simulink model "gmStateSpaceHDL_buck_convert_test1_fixpt"  (R2025a)
settings: Solver=FixedStepAuto  StartTime=0.0  StopTime=0.0005  FixedStep=25e-9  RelTol=1e-3  AbsTol=1e-3
InitFcn:
  | load('C:\Users\bensa\Desktop\PI3_FPGA_BuckConverter\sschdl\buck_convert_test1\stateSpaceParameters.mat');
model workspace (MAT data in the model file):
  NoaFutureIOMap{1}.PortName = 'rst'
  NoaFutureIOMap{1}.PortType = 'Inport'
  NoaFutureIOMap{1}.DataType = 'uint32'
  NoaFutureIOMap{1}.IOInterface = 'AXI4-Lite'
  NoaFutureIOMap{1}.IOInterfaceMapping = 'x"100"'
  NoaFutureIOMap{2}.PortName = 'duty_open_loop'
  NoaFutureIOMap{2}.PortType = 'Inport'
  NoaFutureIOMap{2}.DataType = 'uint32'
  NoaFutureIOMap{2}.IOInterface = 'AXI4-Lite'
  NoaFutureIOMap{2}.IOInterfaceMapping = 'x"104"'
  NoaFutureIOMap{3}.PortName = 'freq'
  NoaFutureIOMap{3}.PortType = 'Inport'
  NoaFutureIOMap{3}.DataType = 'uint32'
  NoaFutureIOMap{3}.IOInterface = 'AXI4-Lite'
  NoaFutureIOMap{3}.IOInterfaceMapping = 'x"108"'
  NoaFutureIOMap{4}.PortName = 'en'
  NoaFutureIOMap{4}.PortType = 'Inport'
  NoaFutureIOMap{4}.DataType = 'uint32'
  NoaFutureIOMap{4}.IOInterface = 'AXI4-Lite'
  NoaFutureIOMap{4}.IOInterfaceMapping = 'x"10C"'
  NoaFutureIOMap{5}.PortName = 'mode_controller'
  NoaFutureIOMap{5}.PortType = 'Inport'
  NoaFutureIOMap{5}.DataType = 'uint32'
  NoaFutureIOMap{5}.IOInterface = 'AXI4-Lite'
  NoaFutureIOMap{5}.IOInterfaceMapping = 'x"110"'
  NoaFutureIOMap{6}.PortName = 'vout_ref'
  NoaFutureIOMap{6}.PortType = 'Inport'
  NoaFutureIOMap{6}.DataType = 'uint32'
  NoaFutureIOMap{6}.IOInterface = 'AXI4-Lite'
  NoaFutureIOMap{6}.IOInterfaceMapping = 'x"114"'
  NoaFutureIOMap{7}.PortName = 'vin'
  NoaFutureIOMap{7}.PortType = 'Outport'
  NoaFutureIOMap{7}.DataType = 'sfix32_En27'
  NoaFutureIOMap{7}.IOInterface = 'DAQ Channel 1 [0:31]'
  NoaFutureIOMap{7}.IOInterfaceMapping = '[0:31]'
  NoaFutureIOMap{8}.PortName = 'vout'
  NoaFutureIOMap{8}.PortType = 'Outport'
  NoaFutureIOMap{8}.DataType = 'sfix32_En27'
  NoaFutureIOMap{8}.IOInterface = 'DAQ Channel 0 [0:31]'
  NoaFutureIOMap{8}.IOInterfaceMapping = '[0:31]'
  NoaFutureIOMap{9}.PortName = 'vout_analog'
  NoaFutureIOMap{9}.PortType = 'Outport'
  NoaFutureIOMap{9}.DataType = 'sfix32_En27'
  NoaFutureIOMap{9}.IOInterface = 'Analog Output 0 [0:31]'
  NoaFutureIOMap{9}.IOInterfaceMapping = '[0:31]'
  NoaFutureIOMap{9}.NoaBlockParameters.SignalMin = '0'
  NoaFutureIOMap{9}.NoaBlockParameters.SignalMax = '12'
  NoaFutureIOMap{9}.NoaBlockParameters.VoltageMin = '0'
  NoaFutureIOMap{9}.NoaBlockParameters.VoltageMax = '4'
  NoaFutureIOMap{9}.NoaBlockParameters.LUT_Signals = '[0          1.2          2.4          3.6          4.8            6          7.2          8.4          9.6         10.8           12]'
  NoaFutureIOMap{9}.NoaBlockParameters.LUT_Values = '[0         0.4         0.8         1.2         1.6           2         2.4         2.8         3.2         3.6           4]'
  NoaFutureIOMap{10}.PortName = 'pwm'
  NoaFutureIOMap{10}.PortType = 'Outport'
  NoaFutureIOMap{10}.DataType = 'ufix32_En29'
  NoaFutureIOMap{10}.IOInterface = 'DAQ Channel 2 [0:31]'
  NoaFutureIOMap{10}.IOInterfaceMapping = '[0:31]'
  NoaFutureIOMap{11}.PortName = 'error_controller'
  NoaFutureIOMap{11}.PortType = 'Outport'
  NoaFutureIOMap{11}.DataType = 'sfix32_En25'
  NoaFutureIOMap{11}.IOInterface = 'DAQ Channel 3 [0:31]'
  NoaFutureIOMap{11}.IOInterfaceMapping = '[0:31]'
values from neighbouring files (symbols this model uses):
  stateSpaceParameters_1 =     [stateSpaceParameters.mat]
libraries: hdlsllib x4, hdlssclib x4, library_AnalogOut x1, simulink x1
CloseFcn:
  | clear stateSpaceParameters_1
settings Model: MinMaxOverflowLogging=MinMaxAndOverflow  FPTRunName=EmbeddedRun1  Creator=bensa  LastModifiedBy=bensa
settings SolverCC: AutoScaleAbsTol=off  AlgebraicLoopSolver=TrustRegion  AutoInsertRateTranBlk=on  MaxZcPerStep=1.0
settings OptimizationCC: BlockReduction=off  ConditionallyExecuteInputs=off  DefaultParameterBehavior=Inlined  InheritOutputTypeSmallerThanSingle=on
settings DebuggingCC: SignalRangeChecking=warning  ArtificialAlgebraicLoopMsg=error  SingleTaskRateTransMsg=error  ParameterOverflowMsg=warning  ParameterUnderflowMsg=warning  UnconnectedInputMsg=warning  UnconnectedOutputMsg=warning  UnconnectedLineMsg=warning  SymbolicDimsDataTypeCodeGenerationDiagnostic=none
settings HardwareCC: ProdBitPerPointer=32.0  ProdBitPerSizeT=32.0  ProdBitPerPtrDiffT=32.0  ProdLargestAtomicFloat=None  ProdIntDivRoundTo=Undefined  ProdEndianess=Unspecified  ProdWordSize=32.0  ProdHWDeviceType=ASIC/FPGA->ASIC/FPGA  TargetBitPerPointer=64.0  TargetBitPerSizeT=64.0  TargetBitPerPtrDiffT=64.0  TargetLongLongMode=on  TargetIntDivRoundTo=Zero  TargetEndianess=LittleEndian  TargetWordSize=64.0  TargetHWDeviceType=Custom Processor->MATLAB Host Computer  ProdEqTarget=off
settings ModelReferenceCC: EnableRefExpFcnMdlSchedulingChecks=on
settings SFSimCC: CustomCodeUndefinedFunction=UseInterfaceOnly
settings RTWCC: GPUComputeCapability=3.5  DLArmComputeVersion=19.05
settings SimscapeCC: SimscapeLogType=all  SimscapeLogSimulationStatistics=on  SimscapeLogDataHistory=10000.0

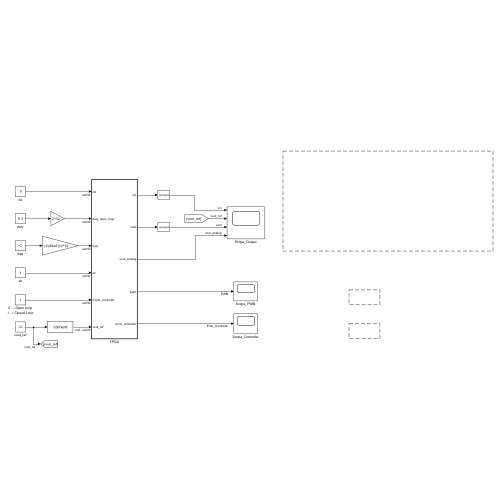
[thumbnail: Simulink's stored preview of the top-level diagram]
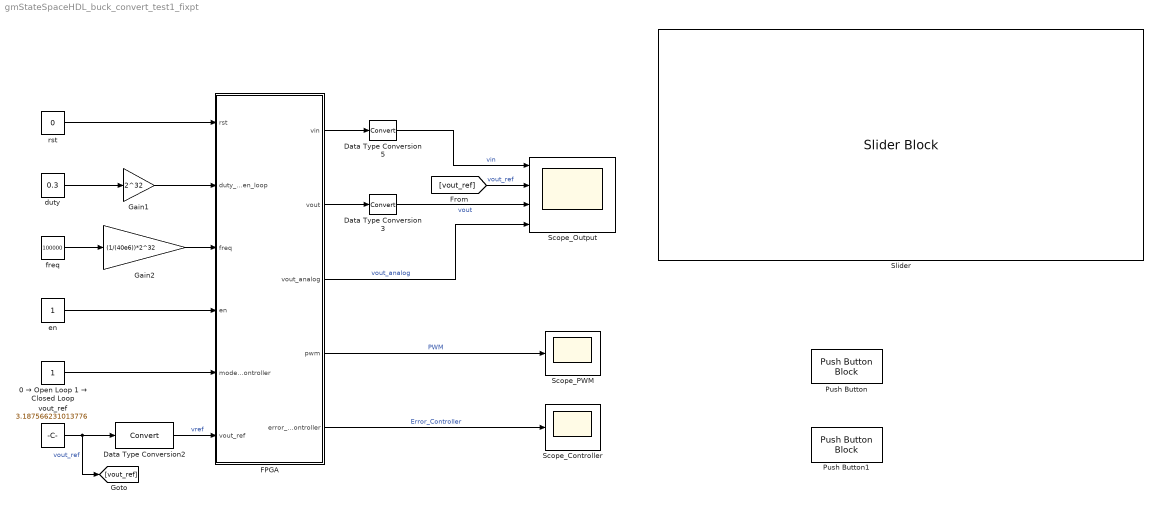
== system gmStateSpaceHDL_buck_convert_test1_fixpt ==
  0 → Open Loop 1 → Closed Loop : Constant  OutDataTypeStr=uint32  SampleTime=25e-9
  Data Type Conversion2 : DataTypeConversion  SaturateOnIntegerOverflow=off  RndMeth=Floor
  Data Type Conversion3 : DataTypeConversion  RndMeth=Nearest  SaturateOnIntegerOverflow=off  LockScale=on
  Data Type Conversion5 : DataTypeConversion  RndMeth=Nearest  SaturateOnIntegerOverflow=off  LockScale=on
  FPGA : Subsystem  TreatAsAtomicUnit=on
  Gain1 : Gain  Gain=2^32  OutDataTypeStr=uint32
  Gain2 : Gain  Gain=(1/(40e6))*2^32  OutDataTypeStr=uint32
  Push Button : PushButtonBlock  IconOnColor=[0.0, 0.39215686274509803, 0.0]  IconOffColor=[0.0, 1.0, 0.0]
  Push Button1 : PushButtonBlock  IconOnColor=[0.0, 0.39215686274509803, 0.0]  IconOffColor=[0.0, 1.0, 0.0]
  Scope_Controller : Scope
      settings: ActiveDisplayYMinimum=-13.875  ActiveDisplayYMaximum=24.875  DataLoggingVariableName=ScopeData3
  Scope_Output : Scope  NumInputPorts=4
      settings: ActiveDisplayYMinimum=-1.4999999999999996  ActiveDisplayYMaximum=13.5
  Scope_PWM : Scope
      settings: ActiveDisplayYMinimum=-0.62499999999999989  ActiveDisplayYMaximum=5.625
  Slider : SliderBlock  LabelPosition=Bottom  ScaleMax=12
  duty : Constant  Value=0.3  OutDataTypeStr=double  SampleTime=25e-9
  en : Constant  OutDataTypeStr=uint32  SampleTime=25e-9
  freq : Constant  Value=100000  SampleTime=25e-9
  rst : Constant  Value=0  OutDataTypeStr=uint32  SampleTime=25e-9
  vout_ref : Constant  Value=3.187566231013776  OutDataTypeStr=double  SampleTime=25e-9
  wires:
  rst/1 -> FPGA/1(rst)
  0 → Open Loop 1 → Closed Loop/1 -> FPGA/5(mode_controller)
  duty/1 -> Gain1/1
  en/1 -> FPGA/4(en)
  Gain2/1 -> FPGA/3(freq)
  vout_ref/1 -> [vout_ref], Data Type Conversion2/1  "vout_ref"
  Gain1/1 -> FPGA/2(duty_open_loop)
  Data Type Conversion2/1 -> FPGA/6(vout_ref)  "vref"
  FPGA/1(vin) -> Data Type Conversion5/1
  FPGA/2(vout) -> Data Type Conversion3/1
  Data Type Conversion5/1 -> Scope_Output/1  "vin"
  [vout_ref] -> Scope_Output/2  "vout_ref"
  Data Type Conversion3/1 -> Scope_Output/3  "vout"
  FPGA/3(vout_analog) -> Scope_Output/4  "vout_analog"
  FPGA/5(error_controller) -> Scope_Controller/1  "Error_Controller"
  FPGA/4(pwm) -> Scope_PWM/1  "PWM"
  freq/1 -> Gain2/1

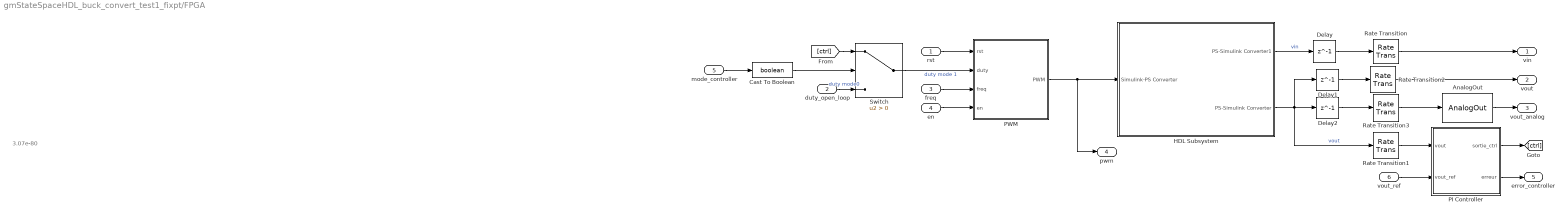
== system gmStateSpaceHDL_buck_convert_test1_fixpt/FPGA ==
  note: 3.07e-80
  rst : Inport  OutDataTypeStr=uint32
  duty_open_loop : Inport  Port=2  OutDataTypeStr=uint32
  freq : Inport  Port=3  OutDataTypeStr=uint32
  en : Inport  Port=4  OutDataTypeStr=uint32
  mode_controller : Inport  Port=5  OutDataTypeStr=uint32
  vout_ref : Inport  Port=6  OutDataTypeStr=uint32
  AnalogOut : library_AnalogOut/AnalogOut  SignalMin=0  SignalMax=12  VoltageMin=0  VoltageMax=4
  Cast To Boolean : DataTypeConversion  OutDataTypeStr=boolean  SaturateOnIntegerOverflow=off  RndMeth=Floor
  Delay : Delay  DelayLength=1
  Delay1 : Delay  DelayLength=1
  Delay2 : Delay  DelayLength=1
  HDL Subsystem : Subsystem  DataTypeOverride=Off  MinMaxOverflowLogging=MinMaxAndOverflow
  PI Controller : Subsystem
  PWM : Subsystem
  Rate Transition : RateTransition  OutPortSampleTime=25e-9
  Rate Transition1 : RateTransition
  Rate Transition2 : RateTransition  OutPortSampleTime=25e-9
  Rate Transition3 : RateTransition  OutPortSampleTime=25e-9
  Switch : Switch  Criteria=u2 > Threshold  SaturateOnIntegerOverflow=off  InputSameDT=off
  vin : Outport
  vout : Outport  Port=2
  vout_analog : Outport  Port=3
  pwm : Outport  Port=4
  error_controller : Outport  Port=5
  wires:
  en/1 -> PWM/4(en)
  mode_controller/1 -> Cast To Boolean/1
  rst/1 -> PWM/1(rst)
  freq/1 -> PWM/3(freq)
  Cast To Boolean/1 -> Switch/2
  Switch/1 -> PWM/2(duty)  "duty mode 1"
  PWM/1(PWM) -> pwm/1, HDL Subsystem/1(Simulink-PS Converter)
  HDL Subsystem/1(PS-Simulink Converter1) -> Delay/1  "vin"
  HDL Subsystem/2(PS-Simulink Converter) -> Rate Transition1/1, Delay2/1, Delay1/1  "vout"
  Delay1/1 -> Rate Transition2/1
  Delay/1 -> Rate Transition/1
  Rate Transition2/1 -> vout/1
  Rate Transition/1 -> vin/1
  AnalogOut/1 -> vout_analog/1
  duty_open_loop/1 -> Switch/3  "duty mode0"
  vout_ref/1 -> PI Controller/2(vout_ref)
  PI Controller/2(erreur) -> error_controller/1
  Rate Transition1/1 -> PI Controller/1(vout)
  Delay2/1 -> Rate Transition3/1
  Rate Transition3/1 -> AnalogOut/1
  PI Controller/1(sortie_ctrl) -> [ctrl]
  [ctrl] -> Switch/1

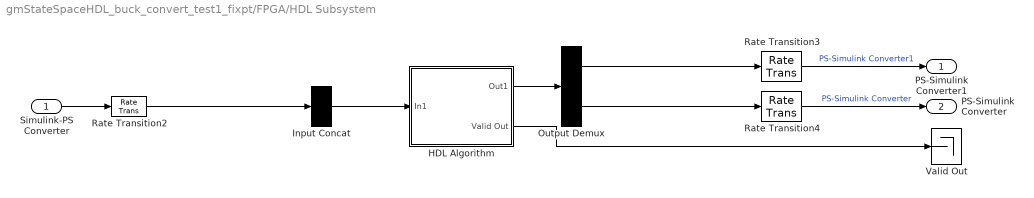
== system gmStateSpaceHDL_buck_convert_test1_fixpt/FPGA/HDL Subsystem ==
  Simulink-PS Converter : Inport  OutDataTypeStr=fixdt(0,32,29)
  HDL Algorithm : Subsystem
  Input Concat : Concatenate  NumInputs=1
  Output Demux : Demux  Outputs=2
  Rate Transition2 : RateTransition  Integrity=off  OutPortSampleTimeOpt=Multiple of input port sample time  OutPortSampleTimeMultiple=1/2
  Rate Transition3 : RateTransition  OutPortSampleTimeOpt=Multiple of input port sample time  OutPortSampleTimeMultiple=2
  Rate Transition4 : RateTransition  OutPortSampleTimeOpt=Multiple of input port sample time  OutPortSampleTimeMultiple=2
  Valid Out : Terminator
  PS-Simulink Converter1 : Outport
  PS-Simulink Converter : Outport  Port=2
  wires:
  Output Demux/2 -> Rate Transition4/1
  Rate Transition3/1 -> PS-Simulink Converter1/1  "PS-Simulink Converter1"
  HDL Algorithm/2(Valid Out) -> Valid Out/1
  Input Concat/1 -> HDL Algorithm/1(In1)
  Output Demux/1 -> Rate Transition3/1
  Simulink-PS Converter/1 -> Rate Transition2/1
  HDL Algorithm/1(Out1) -> Output Demux/1
  Rate Transition4/1 -> PS-Simulink Converter/1  "PS-Simulink Converter"
  Rate Transition2/1 -> Input Concat/1

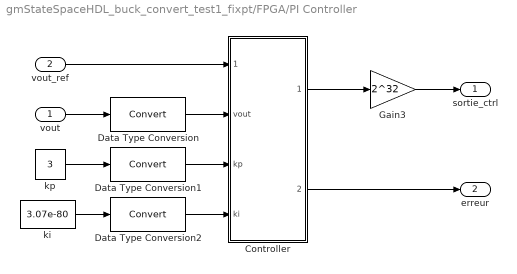
== system gmStateSpaceHDL_buck_convert_test1_fixpt/FPGA/PI Controller ==
  vout : Inport
  vout_ref : Inport  Port=2  OutDataTypeStr=uint32
  Controller : Subsystem
  Data Type Conversion : DataTypeConversion  SaturateOnIntegerOverflow=off  RndMeth=Floor
  Data Type Conversion1 : DataTypeConversion  SaturateOnIntegerOverflow=off  RndMeth=Floor
  Data Type Conversion2 : DataTypeConversion  SaturateOnIntegerOverflow=off  RndMeth=Floor
  Gain3 : Gain  Gain=2^32  OutDataTypeStr=uint32
  ki : Constant  Value=3.07e-80  OutDataTypeStr=double  SampleTime=25e-9
  kp : Constant  Value=3  OutDataTypeStr=double  SampleTime=25e-9
  sortie_ctrl : Outport
  erreur : Outport  Port=2
  wires:
  vout/1 -> Data Type Conversion/1
  Controller/1(sortie_ctrl) -> Gain3/1
  Data Type Conversion1/1 -> Controller/3(kp)
  kp/1 -> Data Type Conversion1/1
  ki/1 -> Data Type Conversion2/1
  vout_ref/1 -> Controller/1(vout_ref)
  Data Type Conversion/1 -> Controller/2(vout)
  Data Type Conversion2/1 -> Controller/4(ki)
  Gain3/1 -> sortie_ctrl/1
  Controller/2(error_ctrl) -> erreur/1

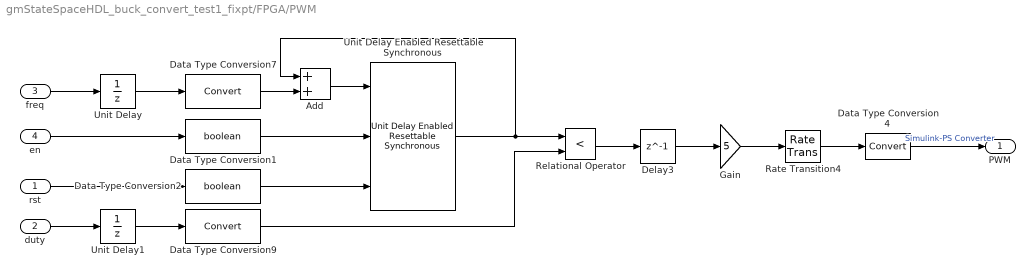
== system gmStateSpaceHDL_buck_convert_test1_fixpt/FPGA/PWM ==
  rst : Inport  OutDataTypeStr=uint32
  duty : Inport  Port=2  OutDataTypeStr=uint32
  freq : Inport  Port=3  OutDataTypeStr=uint32
  en : Inport  Port=4  OutDataTypeStr=uint32
  Add : Sum  OutDataTypeStr=uint32  AccumDataTypeStr=uint32
  Data Type Conversion1 : DataTypeConversion  OutDataTypeStr=boolean  SaturateOnIntegerOverflow=off  RndMeth=Floor
  Data Type Conversion2 : DataTypeConversion  OutDataTypeStr=boolean  SaturateOnIntegerOverflow=off  RndMeth=Floor
  Data Type Conversion4 : DataTypeConversion  RndMeth=Nearest  SaturateOnIntegerOverflow=off
  Data Type Conversion7 : DataTypeConversion  SaturateOnIntegerOverflow=off  RndMeth=Floor
  Data Type Conversion9 : DataTypeConversion  SaturateOnIntegerOverflow=off  RndMeth=Floor
  Delay3 : Delay  DelayLength=1
  Gain : Gain  Gain=5
  Rate Transition4 : RateTransition  OutPortSampleTime=5e-08
  Relational Operator : RelationalOperator  Operator=<  OutDataTypeStr=boolean  RndMeth=Simplest  InputSameDT=off
  Unit Delay : UnitDelay  SampleTime=-1  HasFrameUpgradeWarning=on
  Unit Delay Enabled Resettable Synchronous : hdlsllib/Discrete/Unit Delay Enabled Resettable Synchronous  InitialCondition=0.0  SampleTime=-1
  Unit Delay1 : UnitDelay  SampleTime=-1  HasFrameUpgradeWarning=on
  PWM : Outport
  wires:
  Rate Transition4/1 -> Data Type Conversion4/1
  en/1 -> Data Type Conversion1/1
  Data Type Conversion1/1 -> Unit Delay Enabled Resettable Synchronous/2
  Unit Delay/1 -> Data Type Conversion7/1
  Data Type Conversion7/1 -> Add/2
  Gain/1 -> Rate Transition4/1
  Delay3/1 -> Gain/1
  Data Type Conversion2/1 -> Unit Delay Enabled Resettable Synchronous/3
  Add/1 -> Unit Delay Enabled Resettable Synchronous/1
  freq/1 -> Unit Delay/1
  Unit Delay Enabled Resettable Synchronous/1 -> Add/1, Relational Operator/1
  Unit Delay1/1 -> Data Type Conversion9/1
  rst/1 -> Data Type Conversion2/1
  Data Type Conversion9/1 -> Relational Operator/2
  Relational Operator/1 -> Delay3/1
  duty/1 -> Unit Delay1/1
  Data Type Conversion4/1 -> PWM/1  "Simulink-PS Converter"

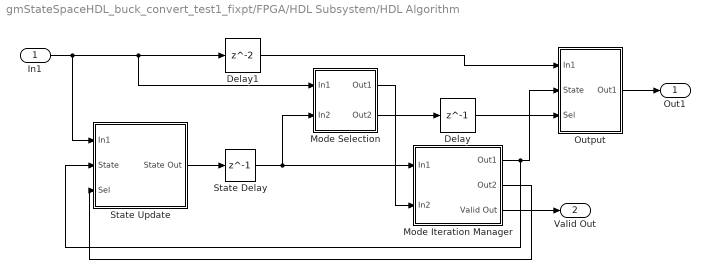
== system gmStateSpaceHDL_buck_convert_test1_fixpt/FPGA/HDL Subsystem/HDL Algorithm ==
  In1 : Inport  OutDataTypeStr=fixdt(0,32,29)
  Delay : Delay  DelayLength=1
  Delay1 : Delay
  Mode Iteration Manager : Subsystem
  Mode Selection : Subsystem
  Output : Subsystem
  State Delay : Delay  DelayLength=1  InitialCondition=single(stateSpaceParameters_1.X0)
  State Update : Subsystem
  Out1 : Outport  VectorParamsAs1DForOutWhenUnconnected=off
  Valid Out : Outport  Port=2  VectorParamsAs1DForOutWhenUnconnected=off
  wires:
  In1/1 -> Mode Selection/1(In1), Delay1/1, State Update/1(In1)
  State Update/1(State Out) -> State Delay/1
  Delay1/1 -> Output/1(In1)
  Mode Selection/2(Out2) -> Delay/1
  State Delay/1 -> Mode Iteration Manager/1(In1), Mode Selection/2(In2)
  Mode Selection/1(Out1) -> Mode Iteration Manager/2(In2)
  Delay/1 -> Output/3(Sel)
  Mode Iteration Manager/1(Out1) -> State Update/2(State), Output/2(State)
  Mode Iteration Manager/2(Out2) -> State Update/3(Sel)
  Mode Iteration Manager/3(Valid Out) -> Valid Out/1
  Output/1(Out1) -> Out1/1

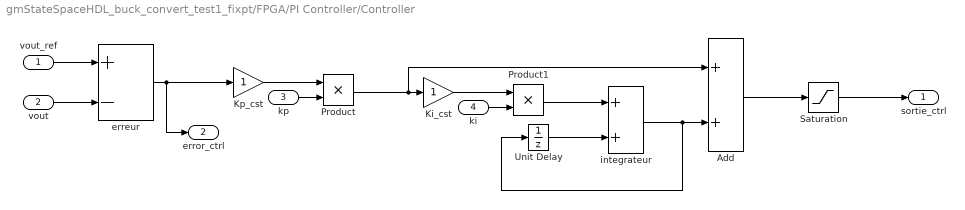
== system gmStateSpaceHDL_buck_convert_test1_fixpt/FPGA/PI Controller/Controller ==
  vout_ref : Inport
  vout : Inport  Port=2
  kp : Inport  Port=3
  ki : Inport  Port=4
  Add : Sum  OutDataTypeStr=fixdt(1,32,25)  AccumDataTypeStr=fixdt(1,32,25)
  Ki_cst : Gain  OutDataTypeStr=fixdt(1,32,25)
  Kp_cst : Gain  OutDataTypeStr=fixdt(1,32,25)
  Product : Product
  Product1 : Product
  Saturation : Saturate  UpperLimit=0.95  LowerLimit=0.05  LinearizeAsGain=off
  Unit Delay : UnitDelay  SampleTime=-1  HasFrameUpgradeWarning=on
  erreur : Sum  Inputs=+-  OutDataTypeStr=fixdt(1,32,25)  AccumDataTypeStr=fixdt(1,32,25)
  integrateur : Sum  OutDataTypeStr=fixdt(1,32,25)  AccumDataTypeStr=fixdt(1,32,25)
  sortie_ctrl : Outport
  error_ctrl : Outport  Port=2
  wires:
  vout/1 -> erreur/2
  vout_ref/1 -> erreur/1
  integrateur/1 -> Unit Delay/1, Add/2
  erreur/1 -> error_ctrl/1, Kp_cst/1
  ki/1 -> Product1/2
  Ki_cst/1 -> Product1/1
  Kp_cst/1 -> Product/1
  Product/1 -> Add/1, Ki_cst/1
  kp/1 -> Product/2
  Product1/1 -> integrateur/1
  Add/1 -> Saturation/1
  Saturation/1 -> sortie_ctrl/1
  Unit Delay/1 -> integrateur/2

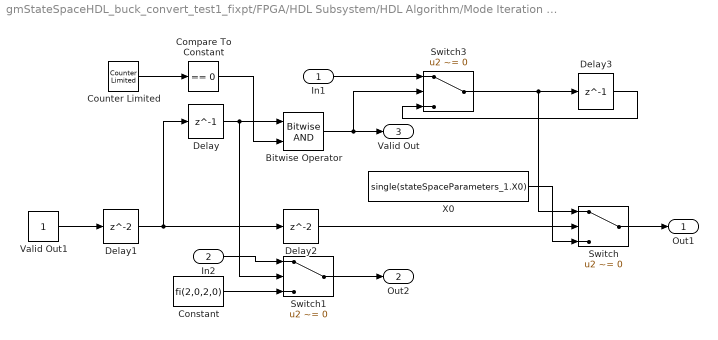
== system gmStateSpaceHDL_buck_convert_test1_fixpt/FPGA/HDL Subsystem/HDL Algorithm/Mode Iteration Manager ==
  In1 : Inport  LockScale=on
  In2 : Inport  Port=2  OutDataTypeStr=fixdt(0,2,0)  LockScale=on
  Bitwise Operator : simulink/Logic and Bit Operations/Bitwise Operator  logicop=AND  UseBitMask=off  NumInputPorts=2  BitMask=bin2dec('11011001')  BitMaskRealWorld=Stored Integer
      settings: LibrarySourceBlock=|
      | hdlsllib/Logic and Bit
      | Operations/Bitwise
      | Operator
  Compare To Constant : hdlsllib/Logic and Bit Operations/Compare To Constant  relop===  const=0  OutDataTypeStr=boolean
  Constant : Constant  Value=fi(2,0,2,0)  SampleTime=2.5e-08  LockScale=on
  Counter Limited : hdlsllib/Sources/Counter Limited  uplimit=1  tsamp=-1
  Delay : Delay  DelayLength=1
  Delay1 : Delay
  Delay2 : Delay
  Delay3 : Delay  DelayLength=1
  Switch : Switch  Criteria=u2 ~= 0  OutDataTypeStr=fixdt(1,32,24)  SaturateOnIntegerOverflow=off  InputSameDT=off
  Switch1 : Switch  Criteria=u2 ~= 0  SaturateOnIntegerOverflow=off  InputSameDT=off  OutDataTypeStr=Inherit: Same as first input
      settings: LockScale=on
  Switch3 : Switch  Criteria=u2 ~= 0  OutDataTypeStr=fixdt(1,32,27)  SaturateOnIntegerOverflow=off  InputSameDT=off
  Valid Out1 : Constant  OutDataTypeStr=boolean  SampleTime=2.5e-08
  X0 : Constant  Value=single(stateSpaceParameters_1.X0)  OutDataTypeStr=fixdt(1,32,27)  SampleTime=2.5e-08
  Out1 : Outport  OutDataTypeStr=fixdt(1,32,24)  VectorParamsAs1DForOutWhenUnconnected=off
  Out2 : Outport  Port=2  VectorParamsAs1DForOutWhenUnconnected=off
  Valid Out : Outport  Port=3  VectorParamsAs1DForOutWhenUnconnected=off
  wires:
  In2/1 -> Switch1/1
  Valid Out1/1 -> Delay1/1
  In1/1 -> Switch3/1
  Counter Limited/1 -> Compare To Constant/1
  Delay/1 -> Switch1/2, Bitwise Operator/1
  Switch3/1 -> Delay3/1, Switch/1
  Delay1/1 -> Delay2/1, Delay/1
  Compare To Constant/1 -> Bitwise Operator/2
  Constant/1 -> Switch1/3
  Bitwise Operator/1 -> Valid Out/1, Switch3/2
  Delay2/1 -> Switch/2
  Switch1/1 -> Out2/1
  X0/1 -> Switch/3
  Delay3/1 -> Switch3/3
  Switch/1 -> Out1/1

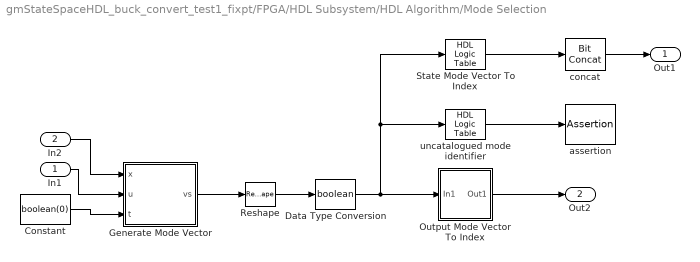
== system gmStateSpaceHDL_buck_convert_test1_fixpt/FPGA/HDL Subsystem/HDL Algorithm/Mode Selection ==
  In1 : Inport  OutDataTypeStr=fixdt(0,32,29)
  In2 : Inport  Port=2  LockScale=on
  Constant : Constant  Value=boolean(0)  SampleTime=2.5e-08
  Data Type Conversion : DataTypeConversion  OutDataTypeStr=boolean  RndMeth=Nearest  SaturateOnIntegerOverflow=off
  Generate Mode Vector : Subsystem  TreatAsAtomicUnit=on  Variant=on
  Output Mode Vector To Index : Subsystem
  Reshape : Reshape
  State Mode Vector To Index : hdlssclib/HDL Logic Table  InputTable=stateSpaceParameters_1.logicTableInput  OutputTable=stateSpaceParameters_1.logicTableOutput
  assertion : Assertion  StopWhenAssertionFail=off
  concat : hdlsllib/Logic and Bit Operations/Bit Concat  numInputs=1
  uncatalogued mode identifier : hdlssclib/HDL Logic Table  InputTable=stateSpaceParameters_1.logicTableInput  OutputTable=ones(size(stateSpaceParameters_1.logicTableOutput,1),1)
  Out1 : Outport  VectorParamsAs1DForOutWhenUnconnected=off  LockScale=on
  Out2 : Outport  Port=2  VectorParamsAs1DForOutWhenUnconnected=off
  wires:
  uncatalogued mode identifier/1 -> assertion/1
  Reshape/1 -> Data Type Conversion/1
  State Mode Vector To Index/1 -> concat/1
  Data Type Conversion/1 -> uncatalogued mode identifier/1, State Mode Vector To Index/1, Output Mode Vector To Index/1(In1)
  Output Mode Vector To Index/1(Out1) -> Out2/1
  concat/1 -> Out1/1
  In2/1 -> Generate Mode Vector/1(x)
  In1/1 -> Generate Mode Vector/2(u)
  Constant/1 -> Generate Mode Vector/3(t)
  Generate Mode Vector/1(vs) -> Reshape/1

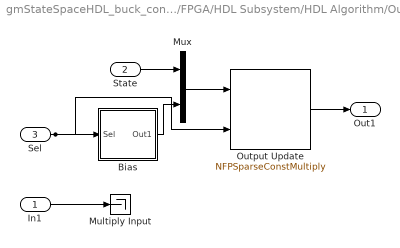
== system gmStateSpaceHDL_buck_convert_test1_fixpt/FPGA/HDL Subsystem/HDL Algorithm/Output ==
  In1 : Inport  OutDataTypeStr=fixdt(0,32,29)
  State : Inport  Port=2  OutDataTypeStr=fixdt(1,32,24)
  Sel : Inport  Port=3  LockScale=on
  Bias : Subsystem
  Multiply Input : Terminator
  Mux : Mux  Inputs=2
  Output Update : hdlssclib/NFPSparseConstMultiply  MatrixSource=Dialog  constMatrix=fi((([stateSpaceParameters_1.Cd repmat(eye(2),[1,1,1])])),1,32,30)  MatrixType=fixdt(1,32,30)  MatrixSize=[1 1]  ColumnIndices=[1]  RowIndices=[1]  PropDataType=fixdt(1,32,27)  defWL=32
  Out1 : Outport  VectorParamsAs1DForOutWhenUnconnected=off
  wires:
  Sel/1 -> Output Update/2, Bias/1(Sel)
  In1/1 -> Multiply Input/1
  State/1 -> Mux/1
  Bias/1(Out1) -> Mux/2
  Mux/1 -> Output Update/1
  Output Update/1 -> Out1/1

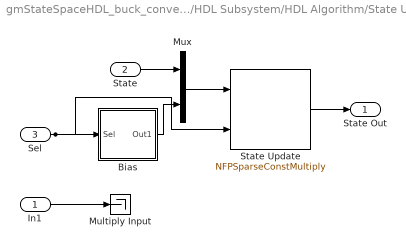
== system gmStateSpaceHDL_buck_convert_test1_fixpt/FPGA/HDL Subsystem/HDL Algorithm/State Update ==
  In1 : Inport  OutDataTypeStr=fixdt(0,32,29)
  State : Inport  Port=2  OutDataTypeStr=fixdt(1,32,24)
  Sel : Inport  Port=3  LockScale=on
  Bias : Subsystem
  Multiply Input : Terminator
  Mux : Mux  Inputs=2
  State Update : hdlssclib/NFPSparseConstMultiply  MatrixSource=Dialog  constMatrix=fi((([stateSpaceParameters_1.Ad repmat(eye(5),[1,1,4])])),1,32,20)  MatrixType=fixdt(1,32,20)  MatrixSize=[1 1]  ColumnIndices=[1]  RowIndices=[1]  PropDataType=fixdt(1,32,18)  defWL=32
  State Out : Outport  VectorParamsAs1DForOutWhenUnconnected=off
  wires:
  Sel/1 -> State Update/2, Bias/1(Sel)
  In1/1 -> Multiply Input/1
  State/1 -> Mux/1
  Mux/1 -> State Update/1
  Bias/1(Out1) -> Mux/2
  State Update/1 -> State Out/1

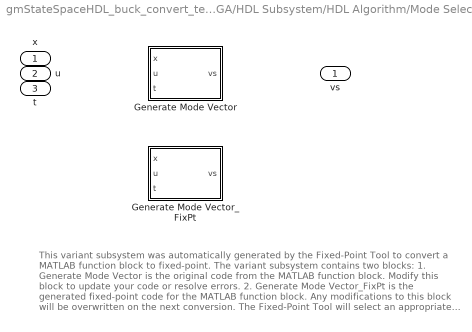
== system gmStateSpaceHDL_buck_convert_test1_fixpt/FPGA/HDL Subsystem/HDL Algorithm/Mode Selection/Generate Mode Vector ==
  note: This variant subsystem was automatically generated by the Fixed-Point Tool to convert a MATLAB function block to fixed-point.
      |
      | The variant subsystem contains two blocks:
      | 1. Generate Mode Vector is the original code from the MATLAB function block. Modify this block to update your code or resolve errors.
      |
      | 2. Generate Mode Vector_FixPt is the generated fixed-point code for the MATLAB function block. Any modifications to this block will be overwritten on the next conversion.
      |
      | The Fixed-Point Tool will select an appropriate variant based on the Model Settings. Learn more.
  x : Inport
  u : Inport  Port=2
  t : Inport  Port=3
  Generate Mode Vector : MATLAB Function  TreatAsAtomicUnit=on  VariantControl=false()
  Generate Mode Vector_FixPt : MATLAB Function  TreatAsAtomicUnit=on  VariantControl=(default)
  vs : Outport

== system gmStateSpaceHDL_buck_convert_test1_fixpt/FPGA/HDL Subsystem/HDL Algorithm/Mode Selection/Output Mode Vector To Index ==
  In1 : Inport
  Index : Constant  Value=fi(0,0,1,0)  SampleTime=2.5e-08  LockScale=on
  Term : Terminator
  Out1 : Outport  VectorParamsAs1DForOutWhenUnconnected=off
  wires:
  In1/1 -> Term/1
  Index/1 -> Out1/1

== system gmStateSpaceHDL_buck_convert_test1_fixpt/FPGA/HDL Subsystem/HDL Algorithm/Output/Bias ==
  Sel : Inport  LockScale=on
  Bias : Constant  Value=single(stateSpaceParameters_1.Y0d)  OutDataTypeStr=fixdt(1,32,24)  SampleTime=2.5e-08
  Terminator : Terminator
  Out1 : Outport  VectorParamsAs1DForOutWhenUnconnected=off
  wires:
  Sel/1 -> Terminator/1
  Bias/1 -> Out1/1

== system gmStateSpaceHDL_buck_convert_test1_fixpt/FPGA/HDL Subsystem/HDL Algorithm/State Update/Bias ==
  Sel : Inport  LockScale=on
  Bias : Constant  Value=single(reshape(stateSpaceParameters_1.F0d,5,4))  OutDataTypeStr=fixdt(1,32,24)  SampleTime=2.5e-08
  Data Type Conversion : DataTypeConversion  OutDataTypeStr=uint32  RndMeth=Nearest  SaturateOnIntegerOverflow=off
  Reshape : Reshape
  Selector : Selector  NumberOfDimensions=2  IndexMode=Zero-based  InputPortWidth=3  IndexOptions=Select all,Index vector (port)  Indices=[1 3]  OutputSizes=1
  Out1 : Outport  VectorParamsAs1DForOutWhenUnconnected=off
  wires:
  Selector/1 -> Reshape/1
  Bias/1 -> Selector/1
  Sel/1 -> Data Type Conversion/1
  Data Type Conversion/1 -> Selector/2
  Reshape/1 -> Out1/1

== matlab function gmStateSpaceHDL_buck_convert_test1_fixpt/FPGA/HDL Subsystem/HDL Algorithm/Mode Selection/Generate Mode Vector/Generate Mode Vector ==
  settings: fimath=fimath('RoundingMethod', 'Floor','OverflowAction', 'Wrap','ProductMode', 'FullPrecision', 'SumMode', 'FullPrecision')
  data: x input; u input; vs output; t input
function vs = compute_modes(x, u, t)

  tmp1 = ((-1.0) .* x(3));
  tmp2 = u(1);

  v1 = (tmp1 > (0.7));
  v2 = (tmp2 > (2.0));

  vs = [v1 v2];

end

== matlab function gmStateSpaceHDL_buck_convert_test1_fixpt/FPGA/HDL Subsystem/HDL Algorithm/Mode Selection/Generate Mode Vector/Generate Mode Vector_FixPt ==
  settings: fimath=fimath('RoundingMethod', 'Floor', 'OverflowAction', 'Wrap', 'ProductMode', 'FullPrecision', 'MaxProductWordLength', 128, 'SumMode', 'FullPrecision', 'MaxSumWordLength', 128)
  data: x input; u input; vs output; t input
%auto-generated
%#codegen
function vs = compute_modes_fixpt(x, u, t)

  fm = get_fimath();
  u = fi(u, 0, 32, 29, fm);

  tmp1 = ((fi(-1.0, 1, 2, 0, fm)) .* x(3));
  tmp2 = fi(u(1), 0, 32, 29, fm);

  v1 = (tmp1 > (fi(0.7, 0, 16, 16, fm)));
  v2 = (tmp2 > (fi(2.0, 0, 2, 0, fm)));

  vs = [v1 v2];

end


function fm = get_fimath()
	fm = fimath('RoundingMethod', 'Floor',...
	     'OverflowAction', 'Wrap',...
	     'ProductMode','FullPrecision',...
	     'MaxProductWordLength', 128,...
	     'SumMode','FullPrecision',...
	     'MaxSumWordLength', 128);
end
